simulink model "arduino_CAN_transmit"  (R2020a)
settings: Solver=FixedStepDiscrete  StartTime=0.0  StopTime=inf  FixedStep=0.01  RelTol=1e-3  EnableMultiTasking=on
libraries: arduinolib x13, simulink x4
settings Model: SimulationMode=external  SILPILModeSetting=veronly  ExtModeTrigDuration=2  Creator=The MathWorks, Inc.  LastModifiedBy=marqu
settings OptimizationCC: EnhancedBackFolding=on  PassReuseOutputArgsThreshold=0  MaxStackSize=64  OptimizeBlockOrder=speed  DifferentSizesBufferReuse=on  OptimizationCustomize=off
settings DebuggingCC: ParameterTunabilityLossMsg=error  SymbolicDimsDataTypeCodeGenerationDiagnostic=none
settings HardwareCC: ProdBitPerInt=16  ProdBitPerPointer=16  ProdBitPerSizeT=16  ProdBitPerPtrDiffT=16  ProdLargestAtomicFloat=None  ProdWordSize=8  ProdHWDeviceType=Atmel->AVR  UseEmbeddedCoderFeatures=off  UseSimulinkCoderFeatures=off
settings SFSimCC: MATLABDynamicMemAlloc=off
settings RTWCC: SystemTargetFile=ert.tlc  HardwareBoard=Arduino Uno  TLCOptions=-aInlineSetEventsForThisBaseRateFcn=TLC_FALSE -aSuppressMultiTaskScheduler=TLC_FALSE -aRateBasedStepFcn=1  TemplateMakefile=ert_default_tmf  GenerateReport=on  Toolchain=Arduino AVR  BuildConfiguration=Faster Runs  LaunchReport=on
settings CodeAppCC: ForceParamTrailComments=on  OperatorAnnotations=on
settings ERTTargetCC: ERTCustomFileBanners=off  SupportContinuousTime=on  SupportNonInlinedSFcns=on  RemoveResetFunc=off  SupportVariableSizeSignals=on  ModelStepFunctionPrototypeControlCompliant=off  ExtModeStaticAllocSize=250

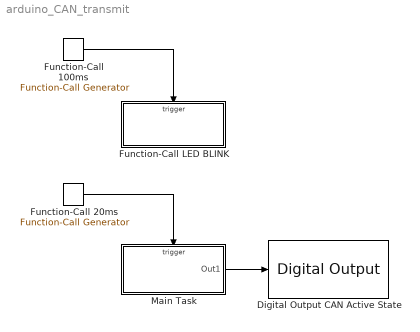
== system arduino_CAN_transmit ==
  "Digital Output CAN Active State " : arduinolib/Digital Output  pinNumber=4  Direction=output  blockPlatform=arduino
  Function-Call 100ms : simulink/Ports & Subsystems/Function-Call Generator  sample_time=0.1  numberOfIterations=1
  Function-Call 20ms : simulink/Ports & Subsystems/Function-Call Generator  sample_time=0.020  numberOfIterations=1
  Function-Call LED BLINK : Subsystem  TreatAsAtomicUnit=on
  Main Task : Subsystem  TreatAsAtomicUnit=on
  wires:
  Function-Call 20ms/1 -> Main Task/Trigger
  Function-Call 100ms/1 -> Function-Call LED BLINK/Trigger
  Main Task/1(Out1) -> "Digital Output CAN Active State "/1

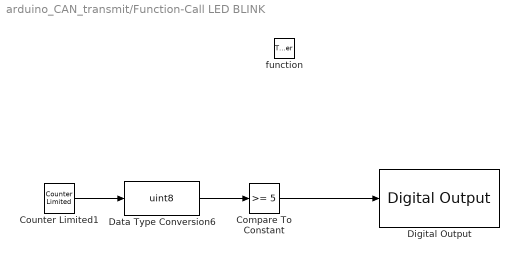
== system arduino_CAN_transmit/Function-Call LED BLINK ==
  function : TriggerPort  TriggerType=function-call  VariantControl=Variant
  Compare To Constant : simulink/Logic and Bit Operations/Compare To Constant  relop=>=  const=5  OutDataTypeStr=boolean
  Counter Limited1 : simulink/Sources/Counter Limited  uplimit=10  tsamp=-1
  Data Type Conversion6 : DataTypeConversion  OutDataTypeStr=uint8
  Digital Output : arduinolib/Digital Output  pinNumber=7  Direction=output  blockPlatform=arduino
  wires:
  Counter Limited1/1 -> Data Type Conversion6/1
  Data Type Conversion6/1 -> Compare To Constant/1
  Compare To Constant/1 -> Digital Output/1

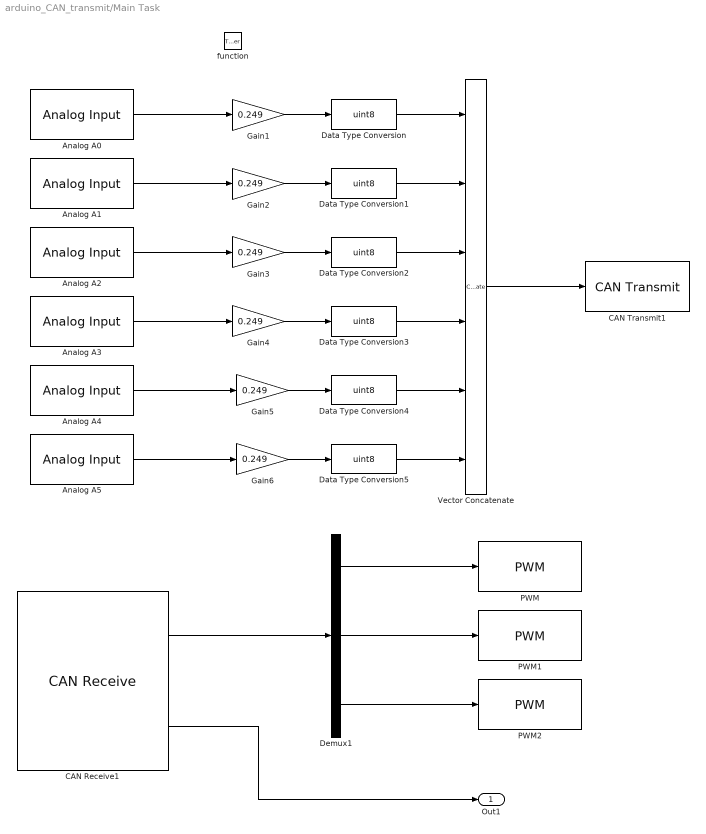
== system arduino_CAN_transmit/Main Task ==
  function : TriggerPort  TriggerType=function-call  VariantControl=Variant
  Analog A0 : arduinolib/Analog Input  pinNumber=0  ReadResultsOnly=off  ConversionTriggerSource=Software  ExternalTriggerType=uint32( 0 )  OutputDataType=uint16  EnableConversionCompleteNotify=off  EnableOuputStatus=off  SampleTime=-1  blockPlatform=arduino
  Analog A1 : arduinolib/Analog Input  pinNumber=1  ReadResultsOnly=off  ConversionTriggerSource=Software  ExternalTriggerType=uint32( 0 )  OutputDataType=uint16  EnableConversionCompleteNotify=off  EnableOuputStatus=off  SampleTime=-1  blockPlatform=arduino
  Analog A2 : arduinolib/Analog Input  pinNumber=2  ReadResultsOnly=off  ConversionTriggerSource=Software  ExternalTriggerType=uint32( 0 )  OutputDataType=uint16  EnableConversionCompleteNotify=off  EnableOuputStatus=off  SampleTime=-1  blockPlatform=arduino
  Analog A3 : arduinolib/Analog Input  pinNumber=3  ReadResultsOnly=off  ConversionTriggerSource=Software  ExternalTriggerType=uint32( 0 )  OutputDataType=uint16  EnableConversionCompleteNotify=off  EnableOuputStatus=off  SampleTime=-1  blockPlatform=arduino
  Analog A4 : arduinolib/Analog Input  pinNumber=4  ReadResultsOnly=off  ConversionTriggerSource=Software  ExternalTriggerType=uint32( 0 )  OutputDataType=uint16  EnableConversionCompleteNotify=off  EnableOuputStatus=off  SampleTime=-1  blockPlatform=arduino
  Analog A5 : arduinolib/Analog Input  pinNumber=5  ReadResultsOnly=off  ConversionTriggerSource=Software  ExternalTriggerType=uint32( 0 )  OutputDataType=uint16  EnableConversionCompleteNotify=off  EnableOuputStatus=off  SampleTime=-1  blockPlatform=arduino
  CAN Receive1 : arduinolib/CAN Receive  outputDataType=Raw data  identifierType=Standard (11-bit identifier)  messageId=100  msgLength=3  SampleTime=inf  outputError=off  outputRemote=off
      settings: SourceProductBaseCode=ARDUINO
  CAN Transmit1 : arduinolib/CAN Transmit  inputDataType=Raw data  BlockingMode_=off  BlockTimeout_=0.05  outputStatus=off  identifierType=Standard (11-bit identifier)  messageId=222  msgLength=6  remoteFrame=off
      settings: SourceProductBaseCode=ARDUINO
  Data Type Conversion{,1..5} (6 alike) : DataTypeConversion  OutDataTypeStr=uint8
  Demux1 : Demux  Outputs=3
  Gain1 : Gain  Gain=0.249
  Gain2 : Gain  Gain=0.249
  Gain3 : Gain  Gain=0.249  OutDataTypeStr=uint8
  Gain4 : Gain  Gain=0.249  OutDataTypeStr=uint16
  Gain5 : Gain  Gain=0.249  OutDataTypeStr=uint16
  Gain6 : Gain  Gain=0.249  OutDataTypeStr=uint16
  PWM : arduinolib/PWM  pinNumber=3  frequencyType=Default  desiredFrequency=490.2  achievableFrequency=490.2
  PWM1 : arduinolib/PWM  pinNumber=5  frequencyType=Default  desiredFrequency=490.2  achievableFrequency=490.2
  PWM2 : arduinolib/PWM  pinNumber=6  frequencyType=Default  desiredFrequency=490.2  achievableFrequency=490.2
  Vector Concatenate : Concatenate  NumInputs=6
  Out1 : Outport
  wires:
  Analog A1/1 -> Gain2/1
  Data Type Conversion4/1 -> Vector Concatenate/5
  Gain6/1 -> Data Type Conversion5/1
  Data Type Conversion2/1 -> Vector Concatenate/3
  Data Type Conversion/1 -> Vector Concatenate/1
  Analog A0/1 -> Gain1/1
  Data Type Conversion5/1 -> Vector Concatenate/6
  Data Type Conversion1/1 -> Vector Concatenate/2
  Analog A2/1 -> Gain3/1
  Gain5/1 -> Data Type Conversion4/1
  Gain1/1 -> Data Type Conversion/1
  Analog A4/1 -> Gain5/1
  Analog A5/1 -> Gain6/1
  Analog A3/1 -> Gain4/1
  Gain2/1 -> Data Type Conversion1/1
  Vector Concatenate/1 -> CAN Transmit1/1
  Gain4/1 -> Data Type Conversion3/1
  Data Type Conversion3/1 -> Vector Concatenate/4
  Gain3/1 -> Data Type Conversion2/1
  CAN Receive1/1 -> Demux1/1
  Demux1/2 -> PWM1/1
  CAN Receive1/2 -> Out1/1
  Demux1/1 -> PWM/1
  Demux1/3 -> PWM2/1
